simulink model "problem3"  (R2024b)
settings: Solver=VariableStepAuto  StartTime=0.0  StopTime=100  RelTol=1e-3
model workspace (MAT data in the model file):
  a_m = 0.7408
  b_m = 0.2592
settings Model: Creator=djd14  LastModifiedBy=djd14

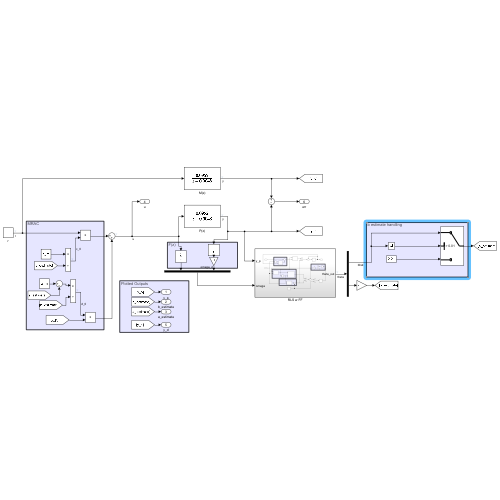
[thumbnail: Simulink's stored preview of the top-level diagram]
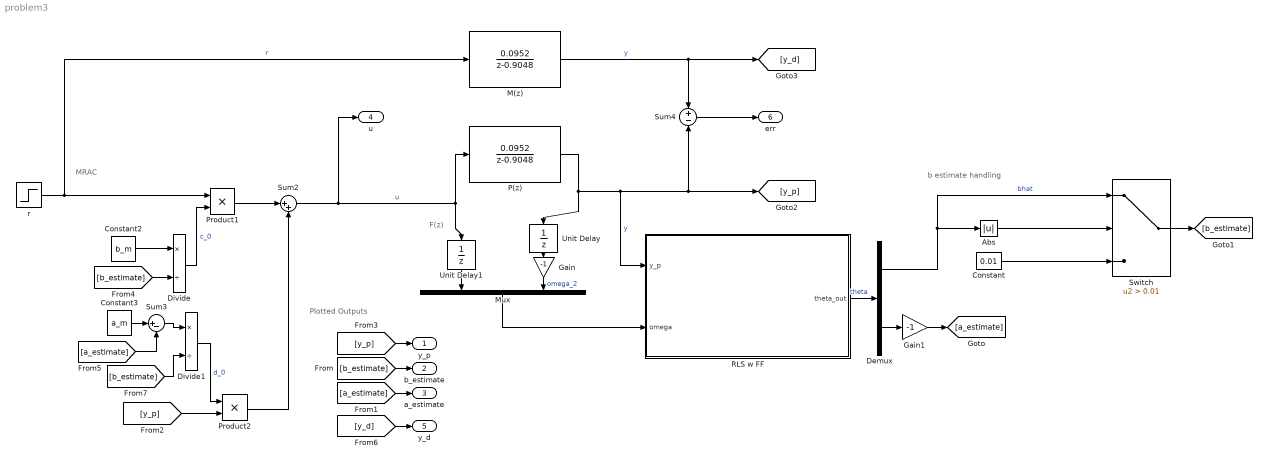
== system problem3 ==
  note: MRAC
  note: b estimate handling
  note: Plotted Outputs
  note: F(z)
  Abs : Abs  SaturateOnIntegerOverflow=off
  Constant : Constant  Value=0.01
  Constant2 : Constant  Value=b_m
  Constant3 : Constant  Value=a_m
  Demux : Demux  Outputs=2
  Divide : Product  Inputs=*/
  Divide1 : Product  Inputs=*/
  Gain : Gain  Gain=-1
  Gain1 : Gain  Gain=-1
  M(z) : DiscreteTransferFcn  Numerator=[0.0952]  Denominator=[1 -0.9048]
  Mux : Mux  Inputs=2
  P(z) : DiscreteTransferFcn  Numerator=[0.0952]  Denominator=[1 -0.9048]
  Product1 : Product
  Product2 : Product
  RLS w FF : Subsystem
  Sum2 : Sum  Inputs=|++
  Sum3 : Sum  Inputs=|+-
  Sum4 : Sum  Inputs=+|-
  Switch : Switch  Criteria=u2 > Threshold  Threshold=0.01  SaturateOnIntegerOverflow=off  InputSameDT=off
  Unit Delay : UnitDelay  SampleTime=-1  HasFrameUpgradeWarning=on
  Unit Delay1 : UnitDelay  SampleTime=-1  HasFrameUpgradeWarning=on
  r : Step  Time=50  Before=1  After=-1  SampleTime=0
  y_p : Outport  SampleTime=1
  b_estimate : Outport  Port=2
  a_estimate : Outport  Port=3
  u : Outport  Port=4
  y_d : Outport  Port=5
  err : Outport  Port=6
  wires:
  Gain/1 -> Mux/2  "omega_2"
  Sum2/1 -> P(z)/1, Unit Delay1/1, u/1  "u"
  RLS w FF/1(theta_out) -> Demux/1  "theta"
  Mux/1 -> RLS w FF/2(omega)
  P(z)/1 -> Sum4/2, [y_p], RLS w FF/1(y_p), Unit Delay/1  "y"
  Demux/2 -> Gain1/1
  Gain1/1 -> [a_estimate]
  [b_estimate] -> b_estimate/1
  [a_estimate] -> a_estimate/1
  r/1 -> M(z)/1, Product1/1  "r"
  [y_p] -> y_p/1
  Demux/1 -> Switch/1, Abs/1  "bhat"
  Abs/1 -> Switch/2
  Switch/1 -> [b_estimate]
  Unit Delay/1 -> Gain/1
  Unit Delay1/1 -> Mux/1
  [b_estimate] -> Divide/2
  Constant2/1 -> Divide/1
  Divide/1 -> Product1/2  "c_0"
  Product1/1 -> Sum2/1
  Constant3/1 -> Sum3/1
  [a_estimate] -> Sum3/2
  Sum3/1 -> Divide1/1
  [y_p] -> Product2/2
  Divide1/1 -> Product2/1  "d_0"
  Product2/1 -> Sum2/2
  M(z)/1 -> [y_d], Sum4/1  "y"
  [y_d] -> y_d/1
  Sum4/1 -> err/1
  [b_estimate] -> Divide1/2
  Constant/1 -> Switch/3

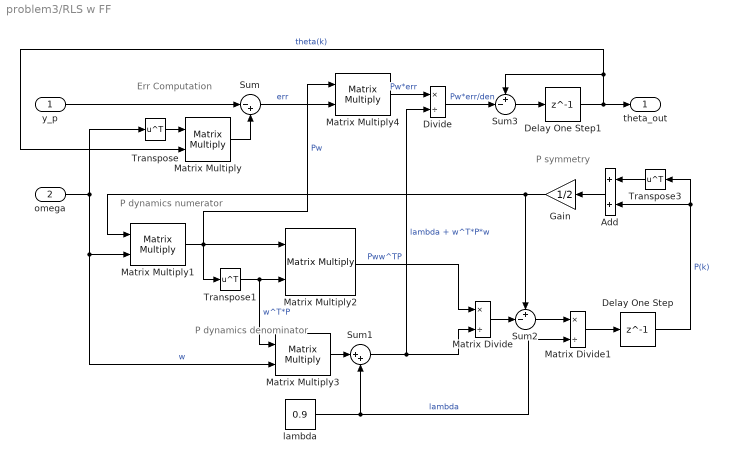
== system problem3/RLS w FF ==
  note: P symmetry
  note: P dynamics denominator
  note: P dynamics numerator
  note: Err Computation
  y_p : Inport
  omega : Inport  Port=2
  Add : Sum
  Delay One Step : Delay  DelayLength=1  InitialCondition=100*eye(2)
  Delay One Step1 : Delay  DelayLength=1  InitialCondition=0
  Divide : Product  Inputs=*/
  Gain : Gain  Gain=1/2
  Matrix Divide : Product  Inputs=*/
  Matrix Divide1 : Product  Inputs=*/
  Matrix Multiply{,1..4} (5 alike) : Product  Multiplication=Matrix(*)
  Sum : Sum  Inputs=|-+
  Sum1 : Sum  Inputs=|++
  Sum2 : Sum  Inputs=+-|
  Sum3 : Sum  Inputs=+-|
  Transpose : Math  Operator=transpose
  Transpose1 : Math  Operator=transpose
  Transpose3 : Math  Operator=transpose
  lambda : Constant  Value=0.9
  theta_out : Outport
  wires:
  omega/1 -> Transpose/1, Matrix Multiply3/2, Matrix Multiply1/2  "w"
  Transpose/1 -> Matrix Multiply/1
  y_p/1 -> Sum/1
  Matrix Multiply/1 -> Sum/2
  Sum/1 -> Matrix Multiply4/2  "err"
  Matrix Multiply1/1 -> Matrix Multiply4/1, Matrix Multiply2/1, Transpose1/1  "Pw"
  Delay One Step/1 -> Transpose3/1, Add/2  "P(k)"
  Matrix Multiply2/1 -> Matrix Divide/1  "Pww^TP"
  Transpose1/1 -> Matrix Multiply3/1, Matrix Multiply2/2  "w^T*P"
  Matrix Multiply3/1 -> Sum1/1
  Sum1/1 -> Divide/2, Matrix Divide/2  "lambda + w^T*P*w"
  Matrix Divide/1 -> Sum2/2
  Sum2/1 -> Matrix Divide1/1
  Matrix Divide1/1 -> Delay One Step/1
  Transpose3/1 -> Add/1
  Add/1 -> Gain/1
  Gain/1 -> Matrix Multiply1/1, Sum2/1
  lambda/1 -> Matrix Divide1/2, Sum1/2  "lambda"
  Sum3/1 -> Delay One Step1/1
  Delay One Step1/1 -> theta_out/1, Matrix Multiply/2, Sum3/1  "theta(k)"
  Matrix Multiply4/1 -> Divide/1  "Pw*err"
  Divide/1 -> Sum3/2  "Pw*err/den"
